simulink model "Progetto_Gruppo21_IZ"  (R2024b)
settings: Solver=FixedStepDiscrete  StartTime=0.0  StopTime=300  FixedStep=0.5  RelTol=1e-3  EnableMultiTasking=on
(part 2 of 2)

== stateflow chart Progetto_Gruppo21_IZ/Chart ==
  state Inizializzazione
    state Stato_Attivo
      state Gestore_logica [parallel]
        settings: executionOrder=1
        state Stato_Operativo
          state Imposta_parametri [parallel]
            settings: executionOrder=2
            state Imposta_output
              en: outputVeneziane = veneziane;
              outputRiscaldamento = rangeRiscaldamento(riscaldamento);
              state Accendi_luci
                en: outputLuci = ON;
              state Spegni_luci
                en: luci = 2;
                outputLuci = OFF;
              (default) -> (junction 594)
              (junction 594) -> Spegni_luci [order 2]
              (junction 594) -> Accendi_luci [order 1] : [luci == 1]
            (default) -> Imposta_output : {veneziane = valoreVeneziane;
                | riscaldamento = valoreRiscaldamento;
                | luci = modLuci;
                | tempo = valoreTemporizzazione;}
          state Stampa_Stato [parallel]
            settings: executionOrder=1
            state Stampa
              en: msgOut = msgAggiornamentoStato(riscaldamento, veneziane, luci, tempo);
            Stampa -> Stampa : after(10, sec)
            (default) -> Stampa : {veneziane = valoreVeneziane;
                | riscaldamento = valoreRiscaldamento;
                | luci = modLuci;
                | tempo = valoreTemporizzazione;}
        state Stato_di_configurazione
          state Uscita_configurazione
            en: msgOut = msgUscita;
            valoreVeneziane = tmpVeneziane;
            valoreRiscaldamento = tmpRiscaldamento;
            valoreTemporizzazione = tmpTemporizzazione;
            modLuci = tmpModLuci;
          state Errore_uscita
            en: msgOut = msgErroreUscita;
          state Stampa_messaggio_configurazione
            en: msgOut = msgConfigurazione;
          state Stato_errore
            en: msgOut = msgErrore;
            ex: msg = "";
          state Salva_configurazione
            en: msgOut = msgSalvataggioConfigurazione;
            tmpVeneziane = valoreVeneziane;
            tmpRiscaldamento = valoreRiscaldamento;
            tmpTemporizzazione = valoreTemporizzazione;
            tmpModLuci = modLuci;
            configurazioneValida = true;
          state Regolazione_veneziane
            state Stampa_iniziale
              en: msgOut = msgRegolazioneVeneziane;
              msg = "";
            state Buffer_veneziane
              en:msg = msg + msgIn;
              msgOut = msgIn;
            state Conferma_valore_veneziane
              en: isValidVeneziane = checkValoreVeneziane(msg);
              msgOut = sprintf('\r\n') + "Controllo valore inserito in corso.";
            state Stampa_valore_veneziane
              en: msgOut = sprintf('\r\n') + "Valore valido impostato: " + msg + " gradi.";
              valoreVeneziane = convertitore(msg);
              ex: msg = "";
            (default) -> Inizializzazione.Stato_Attivo.Gestore_logica.Stato_di_configurazione.Regolazione_veneziane.Stampa_iniziale
            Inizializzazione.Stato_Attivo.Gestore_logica.Stato_di_configurazione.Regolazione_veneziane.Stampa_iniziale -> Buffer_veneziane : [msgInLen > 0]
            Buffer_veneziane -> (junction 313)
            (junction 313) -> Buffer_veneziane [order 2] : [msgInLen > 0]
            (junction 313) -> Conferma_valore_veneziane [order 1] : [msgIn == sprintf('\r')]
            Conferma_valore_veneziane -> (junction 317) : after(1, sec)
            (junction 317) -> Stampa_valore_veneziane [order 1] : [isValidVeneziane]
          state Accensione_luci
            state Stampa_iniziale
              en: msgOut = msgAccensioneLuci;
            state Luci_temporizzate
              state Stampa_iniziale
                en: msgOut = msgConfigurazioneTemporizzazione;
              state Buffer_temporizzazione
                en: msg = msg + msgIn;
                msgOut = msgIn;
              state Conferma_valore_temporizzazione
                en: isValidTemporizzazione = checkValoreTemporizzazione(msg);
                msgOut = sprintf('\r\n') + "Controllo valore inserito in corso.";
              state Stampa_valore_temporizzazione
                en: msgOut = sprintf('\r\n') + "Valore valido impostato: " + msg + " secondi.";
                valoreTemporizzazione = convertitore(msg);
                ex: msg = "";
              (default) -> Inizializzazione.Stato_Attivo.Gestore_logica.Stato_di_configurazione.Accensione_luci.Luci_temporizzate.Stampa_iniziale
              Inizializzazione.Stato_Attivo.Gestore_logica.Stato_di_configurazione.Accensione_luci.Luci_temporizzate.Stampa_iniziale -> Buffer_temporizzazione : [msgInLen > 0]
              Buffer_temporizzazione -> (junction 292)
              (junction 292) -> Buffer_temporizzazione [order 2] : [msgInLen > 0]
              (junction 292) -> Conferma_valore_temporizzazione [order 1] : [msgIn == sprintf('\r')]
              Conferma_valore_temporizzazione -> (junction 282) : after(1, sec)
              (junction 282) -> Stampa_valore_temporizzazione [order 1] : [isValidTemporizzazione]
            state Luci_accese
              en: modLuci = 1;
              msgOut = sprintf('\r\n') + "Impostazione: Luci accese.";
            state Luci_spente
              en: modLuci = 2;
              msgOut = sprintf('\r\n') + "Impostazione: Luci spente.";
            (default) -> Inizializzazione.Stato_Attivo.Gestore_logica.Stato_di_configurazione.Accensione_luci.Stampa_iniziale
            (junction 290) -> (junction 698) [order 3]
            (junction 282) -> (junction 698) [order 2]
            Inizializzazione.Stato_Attivo.Gestore_logica.Stato_di_configurazione.Accensione_luci.Stampa_iniziale -> (junction 290) : [msgInLen > 0]
            (junction 290) -> Luci_accese [order 1] : [msgIn == '1']
            (junction 290) -> Luci_spente [order 2] : [msgIn == '2']
            Luci_spente -> Luci_temporizzate : after(1, sec)
            Luci_accese -> Luci_temporizzate : after(1, sec)
          state Configurazione_riscaldamento
            state Stampa_iniziale
              en: msgOut = msgConfigurazioneRiscaldamento;
              msg = "";
            state Buffer_riscaldamento
              en: msg = msg + msgIn;
              msgOut = msgIn;
            state Conferma_valore_riscaldamento
              en: isValidRiscaldamento = checkValoreRiscaldamento(msg);
              msgOut = sprintf('\r\n') + "Controllo valore inserito in corso.";
            state Stampa_valore_riscaldamento
              en: msgOut = sprintf("\r\n") +"Valore valido impostato: " + msg + " gradi.";
              valoreRiscaldamento = convertitore(msg);
              ex: msg = "";
            (default) -> Inizializzazione.Stato_Attivo.Gestore_logica.Stato_di_configurazione.Configurazione_riscaldamento.Stampa_iniziale
            Inizializzazione.Stato_Attivo.Gestore_logica.Stato_di_configurazione.Configurazione_riscaldamento.Stampa_iniziale -> Buffer_riscaldamento : [msgInLen > 0]
            Buffer_riscaldamento -> (junction 271)
            (junction 271) -> Buffer_riscaldamento [order 2] : [msgInLen > 0]
            (junction 271) -> Conferma_valore_riscaldamento [order 1] : [msgIn == sprintf('\r')]
            Conferma_valore_riscaldamento -> (junction 267) : after(1, sec)
            (junction 267) -> Stampa_valore_riscaldamento [order 1] : [isValidRiscaldamento]
          Stampa_valore_temporizzazione -> (junction 689) : after(1, sec)
          (junction 698) -> (junction 687)
          Stato_di_configurazione -> (junction 529) : [rising(button_config)]
          (default) -> Stampa_messaggio_configurazione : {isValidVeneziane = false;
              | isValidRiscaldamento = false;
              | isValidTemporizzazione = false;
              | msg = "";
              | tmpVeneziane = valoreVeneziane;
              | tmpRiscaldamento = valoreRiscaldamento;
              | tmpTemporizzazione = valoreTemporizzazione;
              | tmpModLuci = modLuci;}
          (junction 687) -> Stato_errore
          Errore_uscita -> (junction 689) : after(1, sec)
          (junction 254) -> (junction 687) [order 6]
          (junction 541) -> Errore_uscita [order 1] : [valoreVeneziane == -1 || valoreRiscaldamento == -1 || modLuci == -1 || valoreTemporizzazione == -1]
          (junction 529) -> Errore_uscita [order 1] : [tmpVeneziane == -1 || tmpRiscaldamento == -1 || tmpModLuci == -1 || tmpTemporizzazione == -1]
          (junction 529) -> Uscita_configurazione [order 2]
          (junction 317) -> (junction 687) [order 2]
          Stampa_valore_veneziane -> (junction 689) : after(1, sec)
          Stampa_messaggio_configurazione -> (junction 254) : [msgInLen > 0]
          Stampa_valore_riscaldamento -> (junction 689) : after(1, sec)
          (junction 689) -> Stampa_messaggio_configurazione
          (junction 254) -> (junction 529) [order 5] : [msgIn == '5']
          (junction 267) -> (junction 687) [order 2]
          Stato_errore -> (junction 689) : after(1, sec)
          (junction 254) -> Configurazione_riscaldamento [order 3] : [msgIn == '3']
          (junction 254) -> (junction 541) [order 4] : [msgIn == '4']
          (junction 541) -> Salva_configurazione [order 2]
          (junction 254) -> Regolazione_veneziane [order 1] : [msgIn == '1']
          (junction 254) -> Accensione_luci [order 2] : [msgIn == '2']
        (default) -> (junction 559)
        (junction 559) -> Stato_di_configurazione [order 1] : [~configurazioneValida]
        (junction 559) -> Stato_Operativo [order 2]
        Uscita_configurazione -> Stato_Operativo : after(1, sec)
        Stato_Operativo -> Stato_di_configurazione : [rising(button_config)]
        Salva_configurazione -> Stato_Operativo : after(1, sec)
      state Led_utente [parallel]
        settings: executionOrder=2
        state Accendi_led
          en: led_utente = ON;
        state Spegni_led
          en: led_utente = OFF;
        (default) -> Accendi_led
        Accendi_led -> Spegni_led : after(0.5, sec)
        Spegni_led -> Accendi_led : after(0.5, sec)
      state Gestione_Pulsanti_Luci [parallel]
        settings: executionOrder=3
        state Stato_di_Attesa
        state Gestore_pulsante_Luci_TMP
          state Caso_luci_accese
            en: luci = 3;
          state Caso_luci_spente
            en: luci = 3;
            outputLuci = ON;
          state Fine_Tempo
            en: luci = 2;
            outputLuci = OFF;
          (default) -> (junction 807)
          (junction 807) -> Inizializzazione.Stato_Attivo.Gestione_Pulsanti_Luci.Gestore_pulsante_Luci_TMP.Caso_luci_spente [order 2]
          (junction 807) -> Inizializzazione.Stato_Attivo.Gestione_Pulsanti_Luci.Gestore_pulsante_Luci_TMP.Caso_luci_accese [order 1] : [luci == 1]
          Inizializzazione.Stato_Attivo.Gestione_Pulsanti_Luci.Gestore_pulsante_Luci_TMP.Caso_luci_accese -> (junction 801)
          Inizializzazione.Stato_Attivo.Gestione_Pulsanti_Luci.Gestore_pulsante_Luci_TMP.Caso_luci_spente -> (junction 801)
          (junction 801) -> Fine_Tempo : after(tempo, sec)
        state Gestore_pulsante_Luci
          state Caso_luci_spente
            en: luci = 1;
            outputLuci = ON;
          state Caso_luci_tmp
            en: luci = 2;
            outputLuci = OFF;
          state Caso_luci_accese
            en: luci = 2;
            outputLuci = OFF;
          (default) -> (junction 798)
          (junction 798) -> Caso_luci_tmp [order 3]
          (junction 798) -> Inizializzazione.Stato_Attivo.Gestione_Pulsanti_Luci.Gestore_pulsante_Luci.Caso_luci_accese [order 1] : [luci == 1]
          (junction 798) -> Inizializzazione.Stato_Attivo.Gestione_Pulsanti_Luci.Gestore_pulsante_Luci.Caso_luci_spente [order 2] : [luci == 2]
          Inizializzazione.Stato_Attivo.Gestione_Pulsanti_Luci.Gestore_pulsante_Luci.Caso_luci_accese -> (junction 799)
          Caso_luci_tmp -> (junction 799)
          Inizializzazione.Stato_Attivo.Gestione_Pulsanti_Luci.Gestore_pulsante_Luci.Caso_luci_spente -> (junction 799)
        (default) -> Stato_di_Attesa
        Stato_di_Attesa -> Gestore_pulsante_Luci [order 1] : [rising(button_Luci) && configurazioneValida]
        Stato_di_Attesa -> Gestore_pulsante_Luci_TMP [order 2] : [rising(button_luci_TMP) && configurazioneValida && valoreTemporizzazione > 0 ]
        (junction 799) -> Stato_di_Attesa
        Fine_Tempo -> Stato_di_Attesa
        Gestore_pulsante_Luci_TMP -> Gestore_pulsante_Luci : [rising(button_Luci)]
    state Stato_Inattivo
      en: msgOut = "Dispositivo non attivo.";
      led_utente = OFF;
      outputVeneziane = 0;
      outputLuci = OFF;
      outputRiscaldamento = 0;
    (default) -> Stato_Inattivo
    Stato_Inattivo -> Stato_Attivo : [rising(button_attivazione)]
    Stato_Attivo -> Stato_Inattivo : [rising(button_attivazione)]{valoreVeneziane = tmpVeneziane;
        |  valoreRiscaldamento = tmpRiscaldamento;
        |  valoreTemporizzazione = tmpTemporizzazione;
        |  modLuci = tmpModLuci;}
  (default) -> Inizializzazione : {valoreVeneziane = -1;
      | valoreRiscaldamento = -1;
      | modLuci = -1;
      | valoreTemporizzazione = -1;
      | configurazioneValida = false;
      | }
  data: outString function_output; outString function_output; outString function_output; outString function_output; outString function_output; outString function_output; val_riscaldamento function_input; val_veneziane function_input; val_luci function_input; val_temporizzazione function_input; outString function_output; outString function_output; outString function_output; outString function_output; result function_output; str function_input; result function_output; str function_input; result function_output; str function_input; val function_input; outRange function_output; str function_input; val function_output; msgOut output string; msgIn input string; msgInLen input; valoreVeneziane local double; valoreRiscaldamento local double; modLuci local double; valoreTemporizzazione local double; msg local string; isValidRiscaldamento local boolean; isValidVeneziane local boolean; isValidTemporizzazione local boolean; tmpVeneziane local double; tmpRiscaldamento local double; tmpTemporizzazione local double; tmpModLuci local double; led_utente output; OFF constant double =0; outputVeneziane output; outputLuci output; button_attivazione input; outputRiscaldamento output; luci local double; riscaldamento local double; tempo local double; veneziane local double; ON constant double =1; button_config input; button_Luci input; button_luci_TMP input; configurazioneValida local boolean
  function outString = msgConfigurazione:
    | function outString = msgConfigurazione
    | %clrscr = sprintf("\033[0;0H\033[2J"); Solo per UART
    | crlf = sprintf('\r\n');
    | 
    | outString = "Configurazione:" + crlf + ...
    |     "1. Regolazione veneziane." + crlf + ...
    |     "2. Accensione luci." + crlf + ...
    |     "3. Configurazione riscaldamento." + crlf + ...
    |     "4. Salva." + crlf + ...;
    |     "5. Esci." + crlf;
    | end
  function outString = msgRegolazioneVeneziane:
    | function outString = msgRegolazioneVeneziane
    | %clrscr = sprintf("\033[0;0H\033[2J"); Solo per UART
    | crlf = sprintf('\r\n');
    | 
    | outString = "Regolazione Veneziane." + crlf + ...
    |    "Inserire un valore da 0 a 180." + crlf + ...
    |    "(Risoluzione di 20)" + crlf;
    | end
  function outString = msgAccensioneLuci:
    | function outString = msgAccensioneLuci
    | %clrscr = sprintf("\033[0;0H\033[2J"); Solo per UART
    | crlf = sprintf('\r\n');
    | 
    | outString = "Configurazione luci." + crlf + ...
    |     "Inserire:" + crlf + ...
    |     "1. Luci accese." + crlf + ...
    |     "2. Luci spente." + crlf;
    | end
  function outString = msgConfigurazioneRiscaldamento:
    | function outString = msgConfigurazioneRiscaldamento
    | %clrscr = sprintf("\033[0;0H\033[2J"); Solo per UART
    | crlf = sprintf('\r\n');
    | 
    | outString = "Configurazione riscaldamento." + crlf + ...
    |     "Inserire un valore compreso tra 16 e 30." + crlf + ...
    |     "(Risoluzione di 1)" + crlf;
    | end
  function outString = msgErroreUscita:
    | function outString = msgErroreUscita
    | %clrscr = sprintf("\033[0;0H\033[2J"); Solo per UART
    | crlf = sprintf('\r\n');
    | 
    | outString = "Configurazione valida non presente." + crlf + ...
    |             "Si prega di inserirne una." + crlf;
    | end
  function outString = msgAggiornamentoStato(val_riscaldamento, val_veneziane, val_luci, val_temporizzazione):
    | function outString = msgAggiornamentoStato(val_riscaldamento, val_veneziane, val_luci, val_temporizzazione)
    | %clrscr = sprintf("\033[0;0H\033[2J"); Solo per UART
    |     crlf = sprintf('\r\n');
    | 
    |     str_veneziane = "Veneziane impostate a " + sprintf('%.1f', val_veneziane) + " gradi.";
    | 
    |     str_luci = "";
    |     if val_luci == 1 || val_luci == 3
    |         str_luci = "Luci accese.";
    |     else
    |         str_luci = "Luci spente.";
    |     end
    |     
    |     str_tempo = "";
    |     if (tempo > 0)
    |        str_tempo = "Temporizzazione luci attiva con tempo: " + sprintf('%.1f', val_temporizzazione) + " secondi.";
    |     else
    |        str_tempo = "Temporizzazione luci non attiva.";
    |     end
    | 
    |     str_riscaldamento = "Riscaldamento impostato a " + sprintf('%.1f', val_riscaldamento) + " gradi.";
    | 
    |     outString = "Stato Operativo:" + crlf + ...
    |        str_veneziane + crlf + ...
    |        str_luci + crlf + ...
    |        str_tempo + crlf + ...
    |        str_riscaldamento + crlf;
    | end
  function outString = msgUscita:
    | function outString = msgUscita
    | %clrscr = sprintf("\033[0;0H\033[2J"); Solo per UART
    | crlf = sprintf('\r\n');
    | 
    | outString = "Uscita in corso." + crlf + ...
    |             "Verranno ripristinate le configurazioni precedenti." + crlf;
    | end
  function outString = msgErrore:
    | function outString = msgErrore
    | %clrscr = sprintf("\033[0;0H\033[2J"); Solo per UART
    | crlf = sprintf('\r\n');
    | 
    | outString = "Valore inserito non valido." + crlf;
    | end
  function outString = msgSalvataggioConfigurazione:
    | function outString = msgSalvataggioConfigurazione
    | %clrscr = sprintf("\033[0;0H\033[2J"); Solo per UART
    | crlf = sprintf('\r\n');
    | 
    | outString = "Configurazione salvata con successo." + crlf;
    | end
  function outString = msgConfigurazioneTemporizzazione:
    | function outString = msgConfigurazioneTemporizzazione
    | %clrscr = sprintf("\033[0;0H\033[2J"); Solo per UART
    | crlf = sprintf('\r\n');
    | 
    | outString = "Configurazione temporizzazione luci." + crlf + ...
    |     "Inserire un valore compreso tra 5 e 30." + crlf + ...
    |     "Inserire 0 per disattivarla." + crlf;
    | end
  function result = checkValoreRiscaldamento(str):
    | function result = checkValoreRiscaldamento(str)
    | 
    |     num = 0;
    |     str = char(str);
    |     for i = 1:length(str)
    |         if str(i) == ' '
    |             break;
    |         end
    |         d = double(str(i)) - 48;
    |         if d < 0 || d > 9
    |             result = false;
    |             return;
    |         end
    |         num = num * 10 + d;
    |     end
    | 
    |     % Verifica validità del numero e range
    |     result = ~isnan(num) && mod(num, 1) == 0 && num >= 16 && num <= 30;
    | end
  function result = checkValoreTemporizzazione(str):
    | function result = checkValoreTemporizzazione(str)
    |   
    |     num = 0;
    |     str = char(str);
    |     isFraction = false;
    |     fractionDivisor = 1;
    | 
    |     for i = 1:length(str)
    |         ch = str(i);
    |         
    |         if ch == ' '
    |             break; 
    |         elseif ch == '.'
    |             if isFraction
    |                 result = false;
    |                 return;
    |             end
    |             isFraction = true;
    |             continue;
    |         end
    |     
    |         d = double(ch) - 48;
    |         if d < 0 || d > 9
    |             result = false;
    |             return;
    |         end
    |     
    |         if ~isFraction
    |             num = num * 10 + d;
    |         else
    |             fractionDivisor = fractionDivisor * 10;
    |             num = num + d / fractionDivisor;
    |         end
    |     end
    | 
    |     % Verifica validità del numero e range
    |     result = ~isnan(num) && ((num >= 5 && num <= 30) || num == 0);
    | end
  function result = checkValoreVeneziane(str):
    | function result = checkValoreVeneziane(str)
    |     
    |     num = 0;
    |     str = char(str);
    |     for i = 1:length(str)
    |         if str(i) == ' '
    |             break;
    |         end
    |         d = double(str(i)) - 48;
    |         if d < 0 || d > 9
    |             result = false;
    |             return;
    |         end
    |         num = num * 10 + d;
    |     end
    | 
    |     % Verifica validità del numero e range
    |     result = ~isnan(num) && mod(num, 20) == 0 && num >= 0 && num <= 180;
    |     
    | end
  function outRange = rangeRiscaldamento(val):
    | function outRange = rangeRiscaldamento(val)
    | 
    |     if val >= 16 && val <= 18
    |             outRange = 0;
    |     elseif val >= 19 && val <= 21
    |             outRange = 1;
    |     elseif val >= 22 && val <= 24
    |             outRange = 2;
    |     elseif val >= 25 && val <= 27
    |             outRange = 3;
    |     elseif val >= 28 && val <= 30
    |             outRange = 4;
    |     else 
    |         outRange = -1
    |     end
    | 
    | end
  function val = convertitore(str):
    | function val = convertitore(str)
    | 
    |     num = 0;
    |     str = char(str);
    |     isFraction = false;
    |     fractionDivisor = 1;
    | 
    |     for i = 1:length(str)
    |         ch = str(i);
    |         
    |         if ch == ' '
    |             break; 
    |         elseif ch == '.'
    |             if isFraction
    |                 val = -1;
    |                 return;
    |             end
    |             isFraction = true;
    |             continue;
    |         end
    |     
    |         d = double(ch) - 48;
    |         if d < 0 || d > 9
    |             val = -1;
    |             return;
    |         end
    |     
    |         if ~isFraction
    |             num = num * 10 + d;
    |         else
    |             fractionDivisor = fractionDivisor * 10;
    |             num = num + d / fractionDivisor;
    |         end
    |     end
    | 
    |     val = num;
    | 
    | end
